simulink model "satellite3"  (R2025b)
settings: Solver=FixedStepAuto  StartTime=0.0  StopTime=100  FixedStep=dt  MinStep=0.0001  RelTol=1e-3
values from neighbouring files (symbols this model uses):
  A_mw = [ ... (first row only)    [init_params.m]
  A_w = [ ... (first row only)    [init_params.m]
  alpha1 = 0.1    [init_params.m]
  alpha2 = 0.1    [init_params.m]
  angle0 = eAR'    [init_params.m]
  area_d = 4    [init_params.m]
  area_m2 = 0.0127    [init_params.m]
  area_s = 2    [init_params.m]
  ARW_deg_per_sqrt_h = 0.01    [init_params.m]
  B_mw = [ ... (first row only)    [init_params.m]
  bat_bias_on = 0    [init_params.m]
  bat_bias_time = 0    [init_params.m]
  bat_bias_value = 0    [init_params.m]
  bat_cap_on = 0    [init_params.m]
  bat_cap_time = 0    [init_params.m]
  bat_cap_value = 1    [init_params.m]
  beta = 0.3    [init_params.m]
  beta1 = 0.01    [init_params.m]
  beta2 = 0.01    [init_params.m]
  bias0_deg_h = 0.01    [init_params.m]
  C_mw = [ ... (first row only)    [init_params.m]
  Cd = 2.2    [init_params.m]
  Cm = 0.01    [init_params.m]
  cmd_comm = 1    [init_params.m]
  comm_allow = 1    [init_params.m]
  cos_g_max = cos(gamma_max)    [init_params.m]
  Cr = 1.2    [init_params.m]
  cT_deg_on = 0    [init_params.m]
  cT_deg_time = 0    [init_params.m]
  cT_deg_value = 1    [init_params.m]
  cT_delay_on = 0    [init_params.m]
  cT_delay_time = 0    [init_params.m]
  cT_delay_value = 0    [init_params.m]
  cT_drop_on = 0    [init_params.m]
  cT_drop_time = 0    [init_params.m]
  cT_drop_value = 0    [init_params.m]
  cT_lock_on = 0    [init_params.m]
  cT_lock_time = 0    [init_params.m]
  d_c = 2e-5    (= 2e-05)    [init_params.m]
  d_f = 2e-5    (= 2e-05)    [init_params.m]
  D_max = 1    [init_params.m]
  D_thr = 0.4    [init_params.m]
  Delta_D = 0.001    [init_params.m]
  dP_th = 0.05    [init_params.m]
  dss_bias_on = 0    [init_params.m]
  dss_bias_time = 0    [init_params.m]
  dss_bias_value = [0;0;0]    [init_params.m]
  dss_delay_on = 0    [init_params.m]
  dss_delay_time = 0    [init_params.m]
  dss_delay_value = 0    [init_params.m]
  dss_drift_max = 0.1    [init_params.m]
  dss_drift_value = [0;0;0]    [init_params.m]
  dss_drop_on = 0    [init_params.m]
  dss_drop_time = 0    [init_params.m]
  dss_drop_value = [1;0;0]    [init_params.m]
  dss_lock_on = 0    [init_params.m]
  dss_lock_time = 0    [init_params.m]
  dt = 0.1    [init_params.m]
  earth_theta0 = 0    [init_params.m]
  epsilon = 0.01    [init_params.m]
  eT_deg_on = 0    [init_params.m]
  eT_deg_time = 0    [init_params.m]
  eT_deg_value = 1    [init_params.m]
  eT_delay_on = 0    [init_params.m]
  eT_delay_time = 0    [init_params.m]
  eT_delay_value = 0    [init_params.m]
  eT_drop_on = 0    [init_params.m]
  eT_drop_time = 0    [init_params.m]
  eT_drop_value = [0;0;0]    [init_params.m]
  eT_lock_on = 0    [init_params.m]
  eT_lock_time = 0    [init_params.m]
  eta = 0.7    [init_params.m]
  eta_buck = 0.9    [init_params.m]
  eta_et = 0.9    [init_params.m]
  eta_sspa = 0.35    [init_params.m]
  eta_twta = 0.35    [init_params.m]
  f = 2.2e9    (= 2200000000)    [init_params.m]
  f_n_hz = 400    [init_params.m]
  fov = 60*pi/180    (= 1.0471975512)    [init_params.m]
  g0 = 9.80665    [init_params.m]
  G0 = 1366.1    [init_params.m]
  G_sspa_dB = 20    [init_params.m]
  G_twta_dB = 20    [init_params.m]
  Gr_dB = 20    [init_params.m]
  Gt_dB = 3    [init_params.m]
  gyro_bias_on = 0    [init_params.m]
  gyro_bias_time = 0    [init_params.m]
  gyro_bias_value = [0;0;0]    [init_params.m]
  gyro_delay_on = 0    [init_params.m]
  gyro_delay_time = 0    [init_params.m]
  gyro_delay_value = 0    [init_params.m]
  gyro_drift_max = 0.1    [init_params.m]
  gyro_drift_value = [0;0;0]    [init_params.m]
  gyro_drop_on = 0    [init_params.m]
  gyro_drop_time = 0    [init_params.m]
  gyro_drop_value = [0;0;0]    [init_params.m]
  gyro_lock_on = 0    [init_params.m]
  gyro_lock_time = 0    [init_params.m]
  H = 50e3    (= 50000)    [init_params.m]
  h_max = Iw * rpm_max * sqrt(6)    [init_params.m]
  h_ref = 400e3    (= 400000)    [init_params.m]
  I_e = 11    [init_params.m]
  I_gate = 0.5    [init_params.m]
  I_triggle = 8    [init_params.m]
  i_w_max = 2    [init_params.m]
  i_w_min = -2    [init_params.m]
  initial_phase = 0    [init_params.m]
  Isp = 220    [init_params.m]
  Isp_et = 1500    [init_params.m]
  Iw = 0.02    [init_params.m]
  J2 = 1.08262668e-3    (= 0.00108262668)    [init_params.m]
  Jx = 10    [init_params.m]
  Jy = 12    [init_params.m]
  Jz = 8    [init_params.m]
  k_a = 4e-4    (= 0.0004)    [init_params.m]
  k_bias1_deg_h_per_C = 1    [init_params.m]
  k_bias2_deg_h_per_C = 0.0    (= 0)    [init_params.m]
  k_h = -0.05    [init_params.m]
  k_sf1_ppm = 1.0    (= 1)    [init_params.m]
  k_sf2_ppm = 0.0    (= 0)    [init_params.m]
  ... (+207 more)
libraries: matrix_library x25, simulink x14, nesl_utility x4, simulink_extras x3, fl_lib x3, ee_lib x1
(part 1 of 5)
settings Model: PauseTimes=2600  PacingRate=0.100000  Creator=NUAA  LastModifiedBy=NUAA
settings SolverCC: InitialStep=0.0001

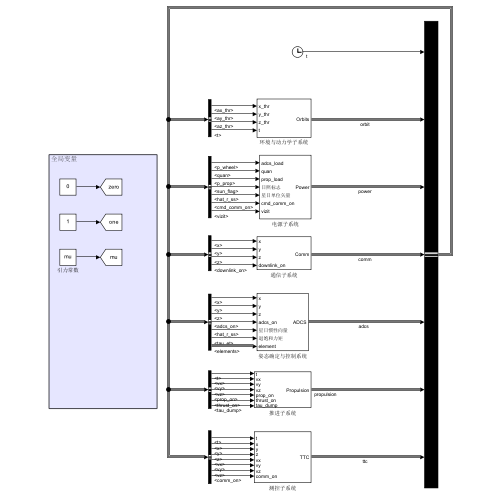
[thumbnail: Simulink's stored preview of the top-level diagram]
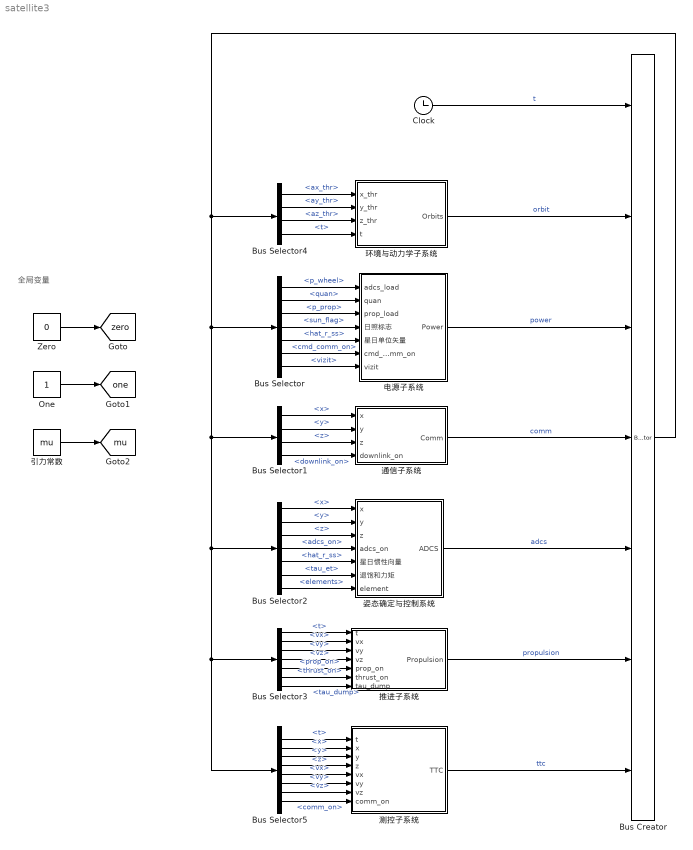
== system satellite3 ==
  note: 全局变量
  Bus Creator : BusCreator  Inputs=7  OutDataTypeStr=Bus: sat
  Bus Selector : BusSelector  OutputSignals=adcs.p_wheel,adcs.quan,propulsion.p_prop,orbit.sun_flag,orbit.hat_r_ss,ttc.cmd_comm_on,ttc.vizit
  Bus Selector1 : BusSelector  OutputSignals=orbit.states.x,orbit.states.y,orbit.states.z,ttc.downlink_on
  Bus Selector2 : BusSelector  OutputSignals=orbit.states.x,orbit.states.y,orbit.states.z,power.adcs_on,orbit.hat_r_ss,propulsion.tau_et,orbit.elements
  Bus Selector3 : BusSelector  OutputSignals=t,orbit.states.vx,orbit.states.vy,orbit.states.vz,power.prop_on,orbit.thrust_on,adcs.tau_dump
  Bus Selector4 : BusSelector  OutputSignals=propulsion.ax_thr,propulsion.ay_thr,propulsion.az_thr,t
  Bus Selector5 : BusSelector  OutputSignals=t,orbit.states.x,orbit.states.y,orbit.states.z,orbit.states.vx,orbit.states.vy,orbit.states.vz,power.comm_on
  Clock : Clock
  One : Constant  OutDataTypeStr=Inherit: Inherit via back propagation
  Zero : Constant  Value=0  OutDataTypeStr=Inherit: Inherit via back propagation
  姿态确定与控制系统 : Subsystem
  引力常数 : Constant  Value=mu  OutDataTypeStr=Inherit: Inherit via back propagation
  推进子系统 : Subsystem
  测控子系统 : Subsystem
  环境与动力学子系统 : Subsystem
  电源子系统 : Subsystem
  通信子系统 : Subsystem
  tag scope: mu=global, one=global, zero=global
  wires:
  Zero/1 -> [zero]
  One/1 -> [one]
  引力常数/1 -> [mu]
  环境与动力学子系统/1(Orbits) -> Bus Creator/2  "orbit"
  电源子系统/1(Power) -> Bus Creator/3  "power"
  Bus Creator/1 -> Bus Selector5/1, Bus Selector3/1, Bus Selector2/1, Bus Selector1/1, Bus Selector/1, Bus Selector4/1
  通信子系统/1(Comm) -> Bus Creator/4  "comm"
  姿态确定与控制系统/1(ADCS) -> Bus Creator/5  "adcs"
  Bus Selector/1 -> 电源子系统/1(adcs_load)  "<p_wheel>"
  Bus Selector/2 -> 电源子系统/2(quan)  "<quan>"
  Bus Selector1/1 -> 通信子系统/1(x)  "<x>"
  Bus Selector1/2 -> 通信子系统/2(y)  "<y>"
  Bus Selector1/3 -> 通信子系统/3(z)  "<z>"
  Bus Selector1/4 -> 通信子系统/4(downlink_on)  "<downlink_on>"
  Bus Selector2/1 -> 姿态确定与控制系统/1(x)  "<x>"
  Bus Selector2/2 -> 姿态确定与控制系统/2(y)  "<y>"
  Bus Selector2/3 -> 姿态确定与控制系统/3(z)  "<z>"
  Clock/1 -> Bus Creator/1  "t"
  Bus Selector2/4 -> 姿态确定与控制系统/4(adcs_on)  "<adcs_on>"
  Bus Selector3/1 -> 推进子系统/1(t)  "<t>"
  Bus Selector3/2 -> 推进子系统/2(vx)  "<vx>"
  Bus Selector3/3 -> 推进子系统/3(vy)  "<vy>"
  推进子系统/1(Propulsion) -> Bus Creator/6  "propulsion"
  Bus Selector/3 -> 电源子系统/3(prop_load)  "<p_prop>"
  Bus Selector3/5 -> 推进子系统/5(prop_on)  "<prop_on>"
  Bus Selector4/1 -> 环境与动力学子系统/1(x_thr)  "<ax_thr>"
  Bus Selector4/2 -> 环境与动力学子系统/2(y_thr)  "<ay_thr>"
  Bus Selector3/4 -> 推进子系统/4(vz)  "<vz>"
  Bus Selector4/3 -> 环境与动力学子系统/3(z_thr)  "<az_thr>"
  Bus Selector/4 -> 电源子系统/4(日照标志)  "<sun_flag>"
  Bus Selector4/4 -> 环境与动力学子系统/4(t)  "<t>"
  Bus Selector/5 -> 电源子系统/5(星日单位矢量)  "<hat_r_ss>"
  Bus Selector3/6 -> 推进子系统/6(thrust_on)  "<thrust_on>"
  Bus Selector2/5 -> 姿态确定与控制系统/5(星日惯性向量)  "<hat_r_ss>"
  测控子系统/1(TTC) -> Bus Creator/7  "ttc"
  Bus Selector5/2 -> 测控子系统/2(x)  "<x>"
  Bus Selector5/3 -> 测控子系统/3(y)  "<y>"
  Bus Selector5/5 -> 测控子系统/5(vx)  "<vx>"
  Bus Selector5/6 -> 测控子系统/6(vy)  "<vy>"
  Bus Selector5/8 -> 测控子系统/8(comm_on)  "<comm_on>"
  Bus Selector5/4 -> 测控子系统/4(z)  "<z>"
  Bus Selector5/1 -> 测控子系统/1(t)  "<t>"
  Bus Selector5/7 -> 测控子系统/7(vz)  "<vz>"
  Bus Selector3/7 -> 推进子系统/7(tau_dump)  "<tau_dump>"
  Bus Selector2/6 -> 姿态确定与控制系统/6(退饱和力矩)  "<tau_et>"
  Bus Selector2/7 -> 姿态确定与控制系统/7(element)  "<elements>"
  Bus Selector/6 -> 电源子系统/6(cmd_comm_on)  "<cmd_comm_on>"
  Bus Selector/7 -> 电源子系统/7(vizit)  "<vizit>"

== system satellite3/姿态确定与控制系统 ==
  x : Inport
  y : Inport  Port=2
  z : Inport  Port=3
  adcs_on : Inport  Port=4
  星日惯性向量 : Inport  Port=5
  退饱和力矩 : Inport  Port=6
  element : Inport  Port=7
  Mux : Mux  Inputs=3
  adcs : BusCreator  Inputs=5  OutDataTypeStr=Bus: adcs
  三轴PD控制器 : Subsystem
  三轴姿态动力学子系统 : Subsystem
      settings: PortSchema="{\"entries\":[{\"content\":{\"sides\":[{\"content\":{\"connectorIds\":[\"In1\",\"In2\",\"In3\"]},\"type\":\"ConnectorPlacement.EquallySpacedRectSide\",\"uuid\":\"b4e63c58-179c-42e3-802d-9c031f031a76\"},{\"content\":{\"connectorIds\":[\"Out1\",\"Out2\",\"Out3\",\"Out4\"],\"side\":\"RIGHT\"},\"type\":\"ConnectorPlacement.EquallySpacedRectSide\",\"uuid\":\"cea4ba66-c4d0-47a6-9ed8-1d5f6e65d5fe\"},{\"content\":{\"connectorIds\":[\"In4\"],\"side\":\"TOP\"},\"type\":\"ConnectorPlacement.EquallySpacedRectSide\",\"uuid\":\"baa71e33-906a-48b3-8a74-2d8b41e12ad9\"},{\"content\":{\"connectorIds\":[\"In5\",\"In6\"],\"side\":\"BOTTOM\"},\"type\":\"ConnectorPlacement.EquallySpacedRectSide\",\"uuid\":\"b6ab8a99-17e4-4d0c-a22a-7f74a164c022\"}]},\"type\":\"ConnectorPlacement.EquallySpacedConnector\",\"uuid\":\"2068c6e4-cb5a-485a-b5bc-bcb903ef601f\"}],\"packageUris\":[\"http://schema.mathworks.com/mf0/Connector/R2020b\"],\"version\":\"1.0\"}"
  向量模长-r_i : Subsystem
  期望四元数 : Constant  Value=QE
  重力梯度力矩 : Subsystem
      settings: PortSchema="{\"entries\":[{\"content\":{\"sides\":[{\"content\":{\"connectorIds\":[\"In1\",\"In2\"]},\"type\":\"ConnectorPlacement.EquallySpacedRectSide\",\"uuid\":\"5e08f9a5-0f22-478e-8a9e-735dc3411939\"},{\"content\":{\"connectorIds\":[\"Out1\",\"Out2\"],\"side\":\"RIGHT\"},\"type\":\"ConnectorPlacement.EquallySpacedRectSide\",\"uuid\":\"e11357c3-d338-4915-97ea-64fb65c259bd\"},{\"content\":{\"side\":\"TOP\"},\"type\":\"ConnectorPlacement.EquallySpacedRectSide\",\"uuid\":\"d2466a98-85a6-4c0d-931a-0ea5053455e9\"},{\"content\":{\"connectorIds\":[\"In3\"],\"side\":\"BOTTOM\"},\"type\":\"ConnectorPlacement.EquallySpacedRectSide\",\"uuid\":\"c799e970-0051-4874-a153-25b8e5bd94de\"}]},\"type\":\"ConnectorPlacement.EquallySpacedConnector\",\"uuid\":\"15237443-cc64-471d-b88e-214b003eddb8\"}],\"packageUris\":[\"http://schema.mathworks.com/mf0/Connector/R2020b\"],\"version\":\"1.0\"}"
  金字塔反作用轮组件 : Subsystem
  ADCS : Outport
  wires:
  三轴PD控制器/1(指令力矩) -> 金字塔反作用轮组件/1(指令力矩)
  金字塔反作用轮组件/1(反作用力矩) -> 三轴姿态动力学子系统/1(反作用力矩)
  三轴姿态动力学子系统/2(解算角速度) -> 三轴PD控制器/2(实际角速率)
  Mux/1 -> 重力梯度力矩/1(r_i)
  y/1 -> 向量模长-r_i/2(u1), Mux/2
  x/1 -> 向量模长-r_i/1(u0), Mux/1
  z/1 -> 向量模长-r_i/3(u2), Mux/3
  向量模长-r_i/1(|u|) -> 重力梯度力矩/2(|r_i|)
  重力梯度力矩/1(T_gg) -> 三轴姿态动力学子系统/3(重力梯度力矩)
  adcs/1 -> ADCS/1
  三轴姿态动力学子系统/1(解算四元数) -> adcs/2, 三轴PD控制器/1(实际四元数)  "quan"
  三轴姿态动力学子系统/3(欧拉数) -> adcs/3  "euler_angle"
  金字塔反作用轮组件/2(轮角动量) -> 三轴姿态动力学子系统/2(轮角动量)
  重力梯度力矩/2(r_o) -> 三轴姿态动力学子系统/5(hat_r_o)
  星日惯性向量/1 -> 三轴姿态动力学子系统/6(hat_ss_i)
  期望四元数/1 -> 三轴PD控制器/3(期望四元数)
  adcs_on/1 -> 三轴PD控制器/4(on)
  金字塔反作用轮组件/3(轮功耗) -> adcs/1  "p_wheel"
  金字塔反作用轮组件/4(wheel) -> adcs/4  "wheel"
  金字塔反作用轮组件/5(指令退饱和力矩) -> adcs/5  "tau_dump"
  退饱和力矩/1 -> 三轴姿态动力学子系统/4(退饱和力矩)
  element/1 -> 重力梯度力矩/3(element)

== system satellite3/推进子系统 ==
  note: 化学推进器 ：主要消耗推进剂，电功耗只体现在阀门/控制器，可设很小常数。
      | 电推进器 ：电功耗很大，推力很小。
  note: 1. 接收供电指令和点火指令。
      | 2. 计算实际推力 T_actual 。
      | 3. 根据 Isp 计算推进剂消耗，积分得到剩余推进剂质量 m_prop 。
      | 4. 用 四元数 把机体系推力方向旋转到惯性系，得到 F_ix, F_iy 。
      | 5. 输出推进加速度 a_thr_x, a_thr_y 给现有 Dynamics，并输出 P_thruster 给现有 Power。
  t : Inport
  vx : Inport  Port=2
  vy : Inport  Port=3
  vz : Inport  Port=4
  prop_on : Inport  Port=5
  thrust_on : Inport  Port=6
  tau_dump : Inport  Port=7
  Add : Sum  Inputs=+++
  Bus Creator : BusCreator  Inputs=5  OutDataTypeStr=Bus: propulsion
  Constant : Constant  Value=m-m0-m0_et
  Divide : Product  Inputs=/*
  Divide1 : Product  Inputs=/*
  Divide2 : Product  Inputs=*/
  Divide3 : Product  Inputs=/*
  Product : Product
  Product1 : Product
  Product2 : Product
  Scope : Scope
      settings: ActiveDisplayYMinimum=0.039953215564435186  ActiveDisplayYMaximum=0.0404210599200833  DataLoggingVariableName=ScopeData26
  Sum : Sum  Inputs=++|
  化推 : Subsystem
  化推功耗 : Switch  Criteria=u2 > Threshold  SaturateOnIntegerOverflow=off  InputSameDT=off
  向量模长-v : Subsystem
  推进功耗 : Constant  Value=P_prop
  电推 : Subsystem
  Propulsion : Outport
  wires:
  prop_on/1 -> 电推/1(prop_on), 化推/1(prop_on)  "电"
  thrust_on/1 -> 化推/2(thrust_on)  "推"
  vy/1 -> Divide1/2, 向量模长-v/2(u2)
  vx/1 -> Divide/2, 向量模长-v/1(u1)
  向量模长-v/1(|u|) -> Divide3/1, Divide/1, Divide1/1
  Constant/1 -> Add/3
  化推/2(left_fuel) -> Add/2
  Add/1 -> Divide2/2
  化推/1(T_act) -> Divide2/1, 化推功耗/2
  Divide/1 -> Product/2
  Divide2/1 -> Scope/1, Product2/1, Product1/1, Product/1
  Divide1/1 -> Product1/2
  推进功耗/1 -> 化推功耗/1
  [zero] -> 化推功耗/3
  Sum/1 -> Bus Creator/2  "p_prop"
  Product/1 -> Bus Creator/3  "ax_thr"
  Product1/1 -> Bus Creator/4  "ay_thr"
  Bus Creator/1 -> Propulsion/1
  vz/1 -> Divide3/2, 向量模长-v/3(u3)
  Product2/1 -> Bus Creator/5  "az_thr"
  Divide3/1 -> Product2/2
  化推功耗/1 -> Sum/2  "p_prop"
  电推/2(left_fuel) -> Add/1
  电推/3(P_et) -> Sum/1  "p_prop"
  tau_dump/1 -> 电推/2(退饱和指令力矩)
  电推/1(tau_et) -> Bus Creator/1  "tau_et"

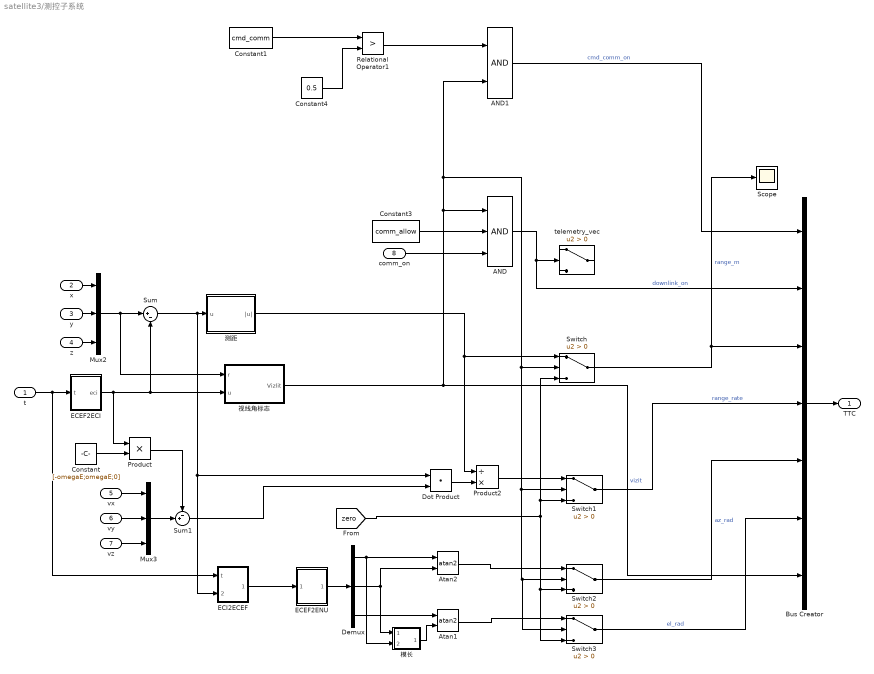
== system satellite3/测控子系统 ==
  t : Inport
  x : Inport  Port=2
  y : Inport  Port=3
  z : Inport  Port=4
  vx : Inport  Port=5
  vy : Inport  Port=6
  vz : Inport  Port=7
  comm_on : Inport  Port=8
  AND : Logic  Inputs=3  AllPortsSameDT=off  OutDataTypeStr=boolean
  AND1 : Logic  AllPortsSameDT=off  OutDataTypeStr=boolean
  Atan1 : Trigonometry  Operator=atan2
  Atan2 : Trigonometry  Operator=atan2
  Bus Creator : BusCreator  Inputs=7  OutDataTypeStr=Bus: ttc
  Constant : Constant  Value=[-omegaE;omegaE;0]
  Constant1 : Constant  Value=cmd_comm
  Constant3 : Constant  Value=comm_allow
  Constant4 : Constant  Value=0.5
  Demux : Demux  Outputs=3
  Dot Product : DotProduct  OutDataTypeStr=Inherit: Inherit via internal rule
  ECEF2ECI : Subsystem
  ECEF2ENU : Subsystem
  ECI2ECEF : Subsystem
  Mux2 : Mux  Inputs=3
  Mux3 : Mux  Inputs=3
  Product : Product
  Product2 : Product  Inputs=/*
  Relational Operator1 : RelationalOperator  Operator=>  OutDataTypeStr=boolean  RndMeth=Simplest  InputSameDT=off
  Scope : Scope
      settings: ActiveDisplayYMinimum=-889765.13346337143  ActiveDisplayYMaximum=8.0078862011703448E+6  DataLoggingVariableName=ScopeData20
  Sum : Sum  Inputs=|+-
  Sum1 : Sum  Inputs=-+|
  Switch{,1..3} (4 alike) : Switch  Criteria=u2 > Threshold  SaturateOnIntegerOverflow=off  InputSameDT=off
  telemetry_vec : Switch  Criteria=u2 > Threshold  SaturateOnIntegerOverflow=off  InputSameDT=off
  模长 : Subsystem
  测距 : Subsystem
  视线角标志 : Subsystem
  TTC : Outport
  wires:
  视线角标志/1(Vizlit) -> Bus Creator/7, AND1/2, Switch3/2, Switch2/2, Switch1/2, Switch/2, AND/1  "vizit"
  测距/1(|u|) -> Switch/1, Product2/1
  Sum1/1 -> Dot Product/2
  Dot Product/1 -> Product2/2
  Product2/1 -> Switch1/1
  Atan2/1 -> Switch2/1
  Constant3/1 -> AND/2
  comm_on/1 -> AND/3
  AND/1 -> Bus Creator/2, telemetry_vec/2  "downlink_on"
  [zero] -> Switch1/3, Switch/3, Switch3/3, Switch2/3
  Switch/1 -> Scope/1, Bus Creator/3  "range_m"
  Switch1/1 -> Bus Creator/4  "range_rate"
  Switch2/1 -> Bus Creator/5  "az_rad"
  Constant1/1 -> Relational Operator1/1
  AND1/1 -> Bus Creator/1  "cmd_comm_on"
  Constant4/1 -> Relational Operator1/2
  Relational Operator1/1 -> AND1/1
  Bus Creator/1 -> TTC/1
  t/1 -> ECI2ECEF/1(t), ECEF2ECI/1(t)
  x/1 -> Mux2/1
  y/1 -> Mux2/2
  z/1 -> Mux2/3
  Mux2/1 -> 视线角标志/1(r), Sum/1
  ECEF2ECI/1(eci) -> Product/1, 视线角标志/2(u), Sum/2
  Sum/1 -> ECI2ECEF/2(In1), Dot Product/1, 测距/1(u)
  vx/1 -> Mux3/1
  vy/1 -> Mux3/2
  vz/1 -> Mux3/3
  Constant/1 -> Product/2
  Mux3/1 -> Sum1/2
  Product/1 -> Sum1/1
  ECI2ECEF/1(ecef) -> ECEF2ENU/1(ecef)
  ECEF2ENU/1(enu) -> Demux/1
  Demux/1 -> 模长/2(u2), Atan2/1
  Demux/2 -> 模长/1(u1), Atan2/2
  Demux/3 -> Atan1/1
  模长/1(|u|) -> Atan1/2
  Atan1/1 -> Switch3/1
  Switch3/1 -> Bus Creator/6  "el_rad"

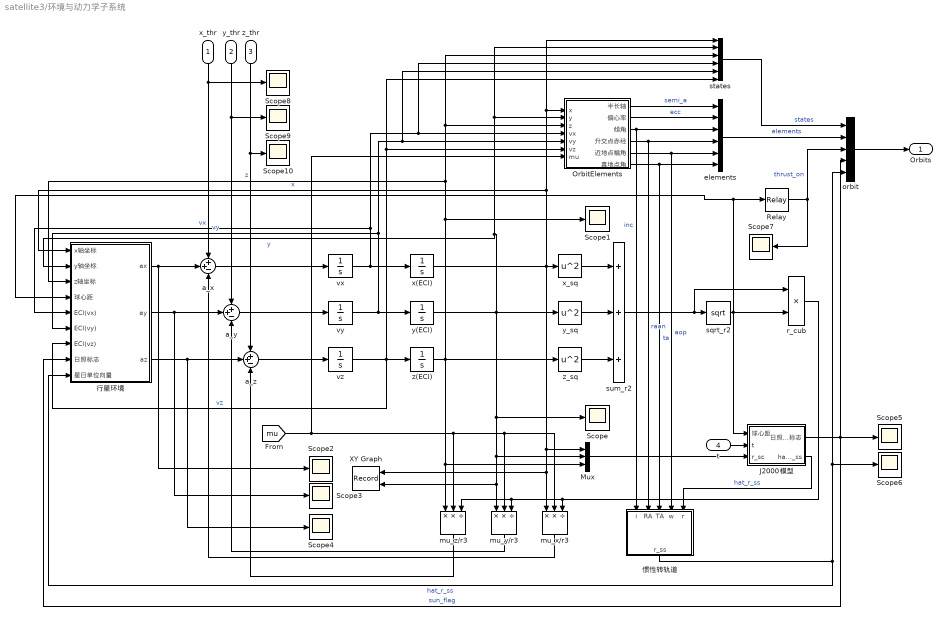
== system satellite3/环境与动力学子系统 ==
  x_thr : Inport
  y_thr : Inport  Port=2
  z_thr : Inport  Port=3
  t : Inport  Port=4
  J2000模型 : Subsystem
  Mux : Mux  Inputs=3
  OrbitElements : Subsystem
  Relay : Relay  OnSwitchValue=r_ref+1e3  OffSwitchValue=r_ref  OnOutputValue=0  OffOutputValue=1  OutDataTypeStr=boolean
  Scope{,1..10} (11 alike) : Scope
      Scope settings: ActiveDisplayYMinimum=-8.9402554358248618E+6  ActiveDisplayYMaximum=8.80467459081228E+6
      Scope1 settings: ActiveDisplayYMinimum=-1  ActiveDisplayYMaximum=1
      Scope10 settings: ActiveDisplayYMinimum=-1  ActiveDisplayYMaximum=1  DataLoggingVariableName=ScopeData25
      Scope2 settings: ActiveDisplayYMinimum=-0.013724283489942623  ActiveDisplayYMaximum=0.013844629667354235  DataLoggingVariableName=ScopeData2
      Scope3 settings: ActiveDisplayYMinimum=-0.013784437757224171  ActiveDisplayYMaximum=0.013784949077631064  DataLoggingVariableName=ScopeData3
      Scope4 settings: ActiveDisplayYMinimum=-5.0430131814522649E-6  ActiveDisplayYMaximum=5.7232220678912172E-7  DataLoggingVariableName=ScopeData4
      Scope5 settings: ActiveDisplayYMinimum=-1  ActiveDisplayYMaximum=1  DataLoggingVariableName=ScopeData10
      Scope6 settings: ActiveDisplayYMinimum=-1  ActiveDisplayYMaximum=1  DataLoggingVariableName=ScopeData17
      Scope7 settings: ActiveDisplayYMinimum=0.88223040201005021  ActiveDisplayYMaximum=1.1253316520100503  DataLoggingVariableName=ScopeData18
      Scope8 settings: ActiveDisplayYMinimum=-1  ActiveDisplayYMaximum=1  DataLoggingVariableName=ScopeData21
      Scope9 settings: ActiveDisplayYMinimum=-1  ActiveDisplayYMaximum=1  DataLoggingVariableName=ScopeData22
  XY Graph : Record  NumPorts=2.0  FileSettingsInternal="{\"entries\":[{\"content\":{\"excelSettings\":{\"content\":{},\"type\":\"Streamout.ExcelSettings\"},\"parquetSettings\":{\"content\":{},\"type\":\"Streamout.ParquetSettings\"}},\"type\":\"Streamout.FileSettingStorage\",\"uuid\":\"\"}],\"packageUris\":[\"http:\\/\\/schema.mathworks.com\\/mf0\\/streamout_blocks\\/R2020a\"],\"version\":\"1.0\"}"  FrameSettings=[0, 0]  Layout=[1 1]  SignalsInternal="{\"entries\":[{\"content\":{\"signals\":[{\"content\":{\"blockPath\":[],\"dimensions\":[1],\"domain\":\"\",\"lineColor\":\"#a2142f\",\"plots\":[ 1 ],\"port\":1,\"sid\":[\"\"],\"signalID\":1,\"signalName\":\"x\"},\"type\":\"RecordBlkView.Signal\",\"uuid\":\"\"},{\"content\":{\"blockPath\":[],\"dimensions\":[1],\"domain\":\"\",\"lineColor\":\"#139fff\",\"plots\":[ 1 ],\"port\":2,\"sid\":[\"\"],\"signalID\":2,\"signalName\":\"y\"},\"type\":\"RecordBlkView.Signal\",\"uuid\":\"\"}]},\"type\":\"RecordBlkView.InputSignals\",\"uuid\":\"\"}],\"packageUris\":[\"http:\\/\\/schema.mathworks.com\\/mf0\\/streamout_blocks\\/R2020a\"],\"version\":\"1.0\"}"  VisualizationBindings="{\"xyplotplugin\":{\"info\":[{\"series\":[{\"bindingParametersList\":[{\"parameter\":\"X-Axis\",\"signalID\":1,\"signalName\":\"x\"},{\"parameter\":\"Y-Axis\",\"signalID\":2,\"signalName\":\"y\"}],\"seriesID\":0}],\"subplotID\":1}]}}"  CompatibilityTag=XY
  a_x : Sum  Inputs=++-
  a_y : Sum  Inputs=++-
  a_z : Sum  Inputs=++-
  elements : BusCreator  Inputs=6  OutDataTypeStr=Bus: elements
  mu_x/r3 : Product  Inputs=**/
  mu_y/r3 : Product  Inputs=**/
  mu_z/r3 : Product  Inputs=**/
  orbit : BusCreator  Inputs=5  OutDataTypeStr=Bus: orbit
  r_cub : Product
  sqrt_r2 : Sqrt
  states : BusCreator  Inputs=6  OutDataTypeStr=Bus: states
  sum_r2 : Sum  Inputs=+++
  vx : Integrator  InitialCondition=vx0
  vy : Integrator  InitialCondition=vy0
  vz : Integrator  InitialCondition=vz0
  x(ECI) : Integrator  InitialCondition=x0
  x_sq : Math  Operator=square
  y(ECI) : Integrator  InitialCondition=y0
  y_sq : Math  Operator=square
  z(ECI) : Integrator  InitialCondition=z0
  z_sq : Math  Operator=square
  惯性转轨道 : MATLAB Function  TreatAsAtomicUnit=on
  行星环境 : Subsystem
  Orbits : Outport
  wires:
  vx/1 -> states/4, OrbitElements/4(vx), 行星环境/5(ECI(vx)), x(ECI)/1  "vx"
  vy/1 -> states/5, OrbitElements/5(vy), 行星环境/6(ECI(vy)), y(ECI)/1  "vy"
  vz/1 -> OrbitElements/6(vz), states/6, 行星环境/7(ECI(vz)), z(ECI)/1  "vz"
  y(ECI)/1 -> y_sq/1, states/2, OrbitElements/2(y), 行星环境/2(y轴坐标), XY Graph/2, mu_y/r3/1, Mux/2, Scope/1  "y"
  x_sq/1 -> sum_r2/1
  y_sq/1 -> sum_r2/2
  z_sq/1 -> sum_r2/3
  sum_r2/1 -> r_cub/1, sqrt_r2/1
  sqrt_r2/1 -> 行星环境/4(球心距), Relay/1, J2000模型/1(球心距), r_cub/2
  [mu] -> OrbitElements/7(mu), mu_x/r3/2, mu_y/r3/2, mu_z/r3/2
  r_cub/1 -> mu_x/r3/3, mu_y/r3/3, mu_z/r3/3
  mu_z/r3/1 -> a_z/3
  a_z/1 -> vz/1
  a_y/1 -> vy/1
  mu_y/r3/1 -> a_y/3
  mu_x/r3/1 -> a_x/3
  x(ECI)/1 -> XY Graph/1, mu_x/r3/1, Mux/1, x_sq/1, states/1, OrbitElements/1(x), 行星环境/1(x轴坐标)  "x"
  z(ECI)/1 -> z_sq/1, mu_z/r3/1, Mux/3, 行星环境/3(z轴坐标), states/3, OrbitElements/3(z), Scope1/1  "z"
  行星环境/1(ax) -> a_x/2, Scope2/1
  行星环境/2(ay) -> a_y/2, Scope3/1
  行星环境/3(az) -> a_z/2, Scope4/1
  a_x/1 -> vx/1
  OrbitElements/1(半长轴) -> elements/1  "semi_a"
  OrbitElements/2(偏心率) -> elements/2  "ecc"
  OrbitElements/3(倾角) -> elements/3, 惯性转轨道/1(i)  "inc"
  OrbitElements/4(升交点赤经) -> elements/4, 惯性转轨道/2(RA)  "raan"
  OrbitElements/5(近地点幅角) -> 惯性转轨道/4(w), elements/5  "aop"
  OrbitElements/6(真地点角) -> 惯性转轨道/3(TA), elements/6  "ta"
  elements/1 -> orbit/2  "elements"
  states/1 -> orbit/1  "states"
  orbit/1 -> Orbits/1
  x_thr/1 -> a_x/1, Scope8/1
  y_thr/1 -> Scope9/1, a_y/1
  Relay/1 -> Scope7/1, orbit/3  "thrust_on"
  z_thr/1 -> Scope10/1, a_z/1
  t/1 -> J2000模型/2(t)
  Mux/1 -> J2000模型/3(r_sc)
  J2000模型/1(日照标志) -> Scope5/1, orbit/4, 行星环境/8(日照标志)  "sun_flag"
  惯性转轨道/1(r_ss) -> orbit/5, Scope6/1, 行星环境/9(星日单位向量)  "hat_r_ss"
  J2000模型/2(hat_r_ss) -> 惯性转轨道/5(r)  "hat_r_ss"

== system satellite3/电源子系统 ==
  adcs_load : Inport
  quan : Inport  Port=2
  prop_load : Inport  Port=3
  日照标志 : Inport  Port=4
  星日单位矢量 : Inport  Port=5
  cmd_comm_on : Inport  Port=6
  vizit : Inport  Port=7
  Add : Sum  Inputs=++++
  Scope : Scope  NumInputPorts=3
      settings: ActiveDisplayYMinimum=-17.3265289803657  ActiveDisplayYMaximum=40.84827911882865  DataLoggingVariableName=ScopeData48
  power : BusCreator  Inputs=4  OutDataTypeStr=Bus: power
  充电调节器 : Subsystem
      settings: PortSchema="{\"entries\":[{\"content\":{\"sides\":[{\"content\":{},\"type\":\"ConnectorPlacement.EquallySpacedRectSide\",\"uuid\":\"1ee7afef-72a2-44d7-b1fe-f775c1bd2fb5\"},{\"content\":{\"connectorIds\":[\"In3\"],\"side\":\"RIGHT\"},\"type\":\"ConnectorPlacement.EquallySpacedRectSide\",\"uuid\":\"a705df99-5add-4aef-8a58-2d39c82bf6d7\"},{\"content\":{\"connectorIds\":[\"Out1\"],\"side\":\"TOP\"},\"type\":\"ConnectorPlacement.EquallySpacedRectSide\",\"uuid\":\"759de5c5-d633-4c5d-bf74-673abcd24ad6\"},{\"content\":{\"connectorIds\":[\"In1\",\"In2\"],\"side\":\"BOTTOM\"},\"type\":\"ConnectorPlacement.EquallySpacedRectSide\",\"uuid\":\"f7dc8a63-c562-404b-8603-e7c277e9b032\"}]},\"type\":\"ConnectorPlacement.EquallySpacedConnector\",\"uuid\":\"7ef34a9a-0568-4899-98ec-73e8b4fd5653\"}],\"packageUris\":[\"http://schema.mathworks.com/mf0/Connector/R2020b\"],\"version\":\"1.0\"}"
  太阳能板 : Subsystem
      settings: PortSchema="{\"entries\":[{\"content\":{\"sides\":[{\"content\":{\"connectorIds\":[\"In1\",\"In2\",\"In3\"]},\"type\":\"ConnectorPlacement.EquallySpacedRectSide\",\"uuid\":\"5bc779c2-c30f-4cae-b4e1-f2edac4125bf\"},{\"content\":{\"connectorIds\":[\"Out1\",\"Out2\",\"Out3\"],\"side\":\"RIGHT\"},\"type\":\"ConnectorPlacement.EquallySpacedRectSide\",\"uuid\":\"cdc54232-7dcb-45bf-9570-abbf77ba5ff8\"},{\"content\":{\"connectorIds\":[\"In4\",\"In5\",\"In6\"],\"side\":\"TOP\"},\"type\":\"ConnectorPlacement.EquallySpacedRectSide\",\"uuid\":\"7ae4bd94-3445-4ae2-aeac-bc49ea099582\"},{\"content\":{\"side\":\"BOTTOM\"},\"type\":\"ConnectorPlacement.EquallySpacedRectSide\",\"uuid\":\"0e5ffc09-da69-4730-b459-bd286bf114a0\"}]},\"type\":\"ConnectorPlacement.EquallySpacedConnector\",\"uuid\":\"4dec81bf-3de5-48e4-88d8-77ff2b0205f0\"}],\"packageUris\":[\"http://schema.mathworks.com/mf0/Connector/R2020b\"],\"version\":\"1.0\"}"
  姿态确认与控制功耗 : Subsystem
  平台常开负载功耗 : Constant  Value=P_base
  推进子系统功耗 : Subsystem
  蓄电池组 : Subsystem
      settings: PortSchema="{\"entries\":[{\"content\":{\"sides\":[{\"content\":{},\"type\":\"ConnectorPlacement.EquallySpacedRectSide\",\"uuid\":\"7e7ce6a8-f422-4b44-b417-981bf143e596\"},{\"content\":{\"connectorIds\":[\"Out1\",\"Out2\"],\"side\":\"RIGHT\"},\"type\":\"ConnectorPlacement.EquallySpacedRectSide\",\"uuid\":\"32e18879-bd9f-43be-9339-7cab6907b877\"},{\"content\":{\"connectorIds\":[\"Out3\"],\"side\":\"TOP\"},\"type\":\"ConnectorPlacement.EquallySpacedRectSide\",\"uuid\":\"64b37c81-2d28-4322-9005-45a88751c011\"},{\"content\":{\"connectorIds\":[\"In1\"],\"side\":\"BOTTOM\"},\"type\":\"ConnectorPlacement.EquallySpacedRectSide\",\"uuid\":\"597055be-0b91-4221-a6e9-97960dc29d81\"}]},\"type\":\"ConnectorPlacement.EquallySpacedConnector\",\"uuid\":\"41982541-c784-41b5-be8a-a88d5d627e5c\"}],\"packageUris\":[\"http://schema.mathworks.com/mf0/Connector/R2020b\"],\"version\":\"1.0\"}"
  通信子系统功耗 : Subsystem
  Power : Outport
  wires:
  蓄电池组/1(V_batt) -> 太阳能板/4(V_batt)
  日照标志/1 -> 太阳能板/1(日照标志), 通信子系统功耗/3(sunlit)
  通信子系统功耗/1(comm_on) -> power/3  "comm_on"
  通信子系统功耗/2(通信功耗) -> Add/2, Scope/2
  太阳能板/3(非欠压) -> 通信子系统功耗/4(not_shed), 推进子系统功耗/3(not_shed), 姿态确认与控制功耗/3(not_shed)
  太阳能板/2(负载电流) -> 充电调节器/1(负载电流)
  vizit/1 -> 通信子系统功耗/2(Vizlit)  "vizlit"
  cmd_comm_on/1 -> 通信子系统功耗/5(cmd_comm_on)
  蓄电池组/3(SOC) -> 充电调节器/3(荷电状态), 姿态确认与控制功耗/1(SOC), power/1, 通信子系统功耗/1(SOC), 推进子系统功耗/1(SOC)  "soc"
  蓄电池组/2(电流差) -> 太阳能板/5(电流差)
  adcs_load/1 -> 姿态确认与控制功耗/2(adcs_load)
  prop_load/1 -> 推进子系统功耗/2(prop_load)
  姿态确认与控制功耗/1(adcs_on) -> power/2  "adcs_on"
  姿态确认与控制功耗/2(P_adcs) -> Scope/1, Add/1
  平台常开负载功耗/1 -> Add/4
  推进子系统功耗/2(prop_on) -> power/4  "prop_on"
  推进子系统功耗/1(P_prop) -> Scope/3, Add/3
  power/1 -> Power/1
  Add/1 -> 太阳能板/6(P_load)
  quan/1 -> 太阳能板/2(q)
  星日单位矢量/1 -> 太阳能板/3(星日单位矢量)
  太阳能板/1(蓄电池充电电流) -> 充电调节器/2(太阳能电池电流)
  充电调节器/1(净充电电流) -> 蓄电池组/1(净充电电流)

== system satellite3/通信子系统 ==
  note: 链路功耗加了，发射功耗还未接入
  note: 通信链可用标志
  note: 接收功率
  note: 信噪比
  note: 把姿态误差引入通信天线增益
      | 引入地面站可见性（地球遮挡）
      | 通信成功 → 数据量积分（任务完成度）
      | 通信失败 → 自动进入安全模式
      | 多地面站切换（Switch + 几何判断）
  note: 如果后面想考虑姿态误差，
      | 只需要在Gt上再减一个pointing loss。
  note: 自由空间路径损耗
      | $\text{FSPL(dBW)}=20\log_{10}{(\frac{4\pi r f}{c})}$
  note: 后续可以改成与地面站的距离
  note: 后续可以添加固放和行波管
  x : Inport
  y : Inport  Port=2
  z : Inport  Port=3
  downlink_on : Inport  Port=4
  10dB : Constant
  20 : Gain  Gain=20
  4pi rf/c : Gain  Gain=4*pi*f
  > : RelationalOperator  Operator=>  OutDataTypeStr=boolean  RndMeth=Simplest  InputSameDT=off
  AND : Logic  AllPortsSameDT=off  OutDataTypeStr=boolean
  Add : Sum  Inputs=-+++
  Constant : Constant  Value=R_data
  Integrator : Integrator  LimitOutput=on  UpperSaturationLimit=1e7  LowerSaturationLimit=0
  Log_10 : Math  Operator=log10
  N_dBW : Constant  Value=Noise_dBW
  SSPA : Subsystem
  Sum : Sum  Inputs=|-+
  Switch : Switch  Criteria=u2 > Threshold  SaturateOnIntegerOverflow=off  InputSameDT=off
  TWTA : Subsystem
  comm : BusCreator  Inputs=4  OutDataTypeStr=Bus: comm
  data_downlinked : Scope
      settings: DataLoggingVariableName=ScopeData11
  发射功率 : Constant  Commented=on  Value=Pt_dBW
  向量模长-r : Subsystem
  地面站天线 : Constant  Value=Gr_dB
  星上天线 : Constant  Value=Gt_dB
  Comm : Outport
  wires:
  x/1 -> 向量模长-r/1(u1)
  y/1 -> 向量模长-r/2(u2)
  z/1 -> 向量模长-r/3(u3)
  向量模长-r/1(|u|) -> 4pi rf/c/1
  4pi rf/c/1 -> Log_10/1
  Log_10/1 -> 20/1
  20/1 -> comm/3, Add/1, Sum/2  "FSPL_dB"
  星上天线/1 -> Add/3
  地面站天线/1 -> Add/4
  Add/1 -> comm/4  "Pr_dBW"
  Sum/1 -> comm/2, >/1  "SNR_dB"
  N_dBW/1 -> Sum/1
  10dB/1 -> >/2
  AND/1 -> Switch/2, comm/1  "link_ok"
  >/1 -> AND/2
  comm/1 -> Comm/1
  downlink_on/1 -> TWTA/1(tx_on), SSPA/1(tx_on), AND/1
  SSPA/1(Pt_dBW) -> Add/2
  [zero] -> Switch/3
  Constant/1 -> Switch/1
  Switch/1 -> Integrator/1
  Integrator/1 -> data_downlinked/1

== system satellite3/姿态确定与控制系统/三轴PD控制器 ==
  note: 在 当前实际姿态 基础上进行的旋转 $Q_e$$ ，使得它叠加在 $Q_a$$ 之后，能够达到期望姿态 $Q_d$$ 。
      | $1:Q_a \otimes Q_e=Q_d \\ 2:Q_a^{-1} \otimes (Q_a \otimes Q_e)=Q_a^{-1} \otimes Q_d \\ 3:Q_e = Q_a^{-1} \otimes Q_d \\ 4:Q_e = Q_a^{*} \otimes Q_d$
  note: 姿态误差限幅，防止大误差时控制器给出不合理力矩
  实际四元数 : Inport
  实际角速率 : Inport  Port=2
  期望四元数 : Inport  Port=3
  on : Inport  Port=4
  Demux : Demux
  Mux : Mux  Inputs=3
  Product : Product
  Product1 : Product
  Relay(qe0) : Relay  OffOutputValue=-1
  Scope : Scope
      settings: ActiveDisplayYMinimum=-0.83029524631328933  ActiveDisplayYMaximum=3.1480849645197186  DataLoggingVariableName=ScopeData32
  Sum1 : Sum  Inputs=|+-
  Switch : Switch  Criteria=u2 > Threshold  SaturateOnIntegerOverflow=off  InputSameDT=off
  sign(q0) : Signum
  共轭 : Subsystem
  四元数乘法 : Subsystem
  四元数归一化 : Subsystem
  姿态控制器-微分 : Gain  Gain=Kd
  姿态控制器-比例 : Gain  Gain=Kp
  指令力矩 : Outport
  wires:
  Product/1 -> 姿态控制器-比例/1
  姿态控制器-比例/1 -> Sum1/1
  姿态控制器-微分/1 -> Sum1/2
  期望四元数/1 -> 四元数归一化/1(In1)
  实际四元数/1 -> 共轭/1(u)
  四元数乘法/1(四元数旋转偏差) -> Demux/1
  Demux/1 -> Relay(qe0)/1
  Demux/2 -> Mux/1
  Demux/3 -> Mux/2
  Demux/4 -> Mux/3
  Mux/1 -> Product/2
  Relay(qe0)/1 -> Product/1
  实际角速率/1 -> 姿态控制器-微分/1
  共轭/1(u^-1) -> 四元数乘法/1(Q1)
  on/1 -> Product1/2
  四元数归一化/1(Out1) -> 四元数乘法/2(Q2)
  Sum1/1 -> 指令力矩/1, Product1/1
  Product1/1 -> Scope/1

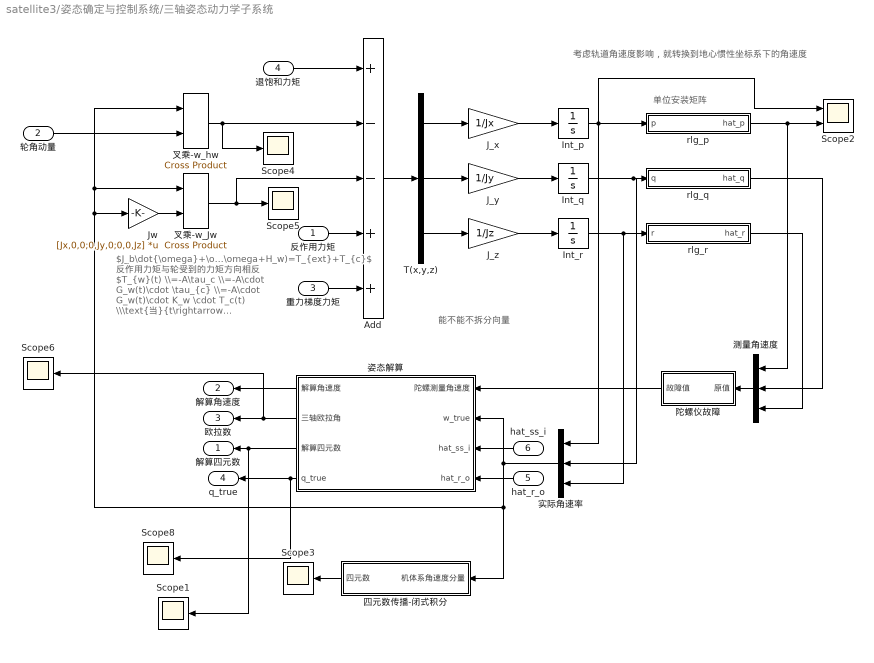
== system satellite3/姿态确定与控制系统/三轴姿态动力学子系统 ==
  note: $J_b\dot{\omega}+\omega\times(J_b\omega+H_w)=T_{ext}+T_{c}$
      | 反作用力矩与轮受到的力矩方向相反
      | $T_{w}(t) \\=-A\tau_c \\=-A\cdot G_w(t)\cdot \tau_{c} \\=-A\cdot G_w(t)\cdot K_w \cdot T_c(t) \\\text{当}{t\rightarrow t_s},G_w(t)=1,T_w(t)=-T_c(t)$
  note: 考虑轨道角速度影响，就转换到地心惯性坐标系下的角速度
  note: 能不能不拆分向量
  note: 单位安装矩阵
  反作用力矩 : Inport
  轮角动量 : Inport  Port=2
  重力梯度力矩 : Inport  Port=3
  退饱和力矩 : Inport  Port=4
  hat_r_o : Inport  Port=5
  hat_ss_i : Inport  Port=6
  Add : Sum  Inputs=+--++
  Int_p : Integrator  InitialCondition=w0(1)  LimitOutput=on  UpperSaturationLimit=p_sat*pi/180  LowerSaturationLimit=-10*pi/180
  Int_q : Integrator  InitialCondition=w0(2)  LimitOutput=on  UpperSaturationLimit=10*pi/180  LowerSaturationLimit=-10*pi/180
  Int_r : Integrator  InitialCondition=w0(3)  LimitOutput=on  UpperSaturationLimit=10*pi/180  LowerSaturationLimit=-10*pi/180
  J_x : Gain  Gain=1/Jx
  J_y : Gain  Gain=1/Jy
  J_z : Gain  Gain=1/Jz
  Jw : Gain  Gain=[Jx,0,0;0,Jy,0;0,0,Jz]  Multiplication=Matrix(K*u)
  Scope{1,3..6,8} (6 alike) : Scope
      Scope1 settings: ActiveDisplayYMinimum=-0.82477001832836239  ActiveDisplayYMaximum=0.987415638960409  DataLoggingVariableName=ScopeData8
      Scope3 settings: ActiveDisplayYMinimum=-0.607859112920923  ActiveDisplayYMaximum=1.0348923894829236  DataLoggingVariableName=ScopeData8
      Scope4 settings: ActiveDisplayYMinimum=-0.00074445474291978057  ActiveDisplayYMaximum=0.00081473788246158054  DataLoggingVariableName=ScopeData23
      Scope5 settings: ActiveDisplayYMinimum=-6.9419152004580546E-8  ActiveDisplayYMaximum=8.6121465383319188E-8  DataLoggingVariableName=ScopeData24
      Scope6 settings: ActiveDisplayYMinimum=-5.13179233941835  ActiveDisplayYMaximum=5.9674363348372523  DataLoggingVariableName=ScopeData31
      Scope8 settings: ActiveDisplayYMinimum=-1.164089564599627  ActiveDisplayYMaximum=1.0182326383526819  DataLoggingVariableName=ScopeData33
  Scope2 : Scope  NumInputPorts=2
      settings: ActiveDisplayYMinimum=-1.1823301841470205E-6  ActiveDisplayYMaximum=2.0642729555703557E-6  DataLoggingVariableName=ScopeData6
  T(x,y,z) : Demux  Outputs=3
  rlg_p : Subsystem
  rlg_q : Subsystem
  rlg_r : Subsystem
  叉乘-w_Jw : matrix_library/Cross Product
  叉乘-w_hw : matrix_library/Cross Product
  四元数传播-闭式积分 : Subsystem
  姿态解算 : Subsystem
  实际角速率 : Mux  Inputs=3
  测量角速度 : Mux  Inputs=3
  陀螺仪故障 : Subsystem
  解算四元数 : Outport
  解算角速度 : Outport  Port=2
  欧拉数 : Outport  Port=3
  q_true : Outport  Port=4
  wires:
  Add/1 -> T(x,y,z)/1
  叉乘-w_hw/1 -> Scope4/1, Add/2
  轮角动量/1 -> 叉乘-w_hw/2
  反作用力矩/1 -> Add/4
  J_z/1 -> Int_r/1
  T(x,y,z)/1 -> J_x/1
  J_y/1 -> Int_q/1
  T(x,y,z)/2 -> J_y/1
  J_x/1 -> Int_p/1
  T(x,y,z)/3 -> J_z/1
  Int_p/1 -> 实际角速率/1, Scope2/1, rlg_p/1(p)
  Int_q/1 -> 实际角速率/2, rlg_q/1(q)
  Int_r/1 -> 实际角速率/3, rlg_r/1(r)
  Jw/1 -> 叉乘-w_Jw/2
  叉乘-w_Jw/1 -> Scope5/1, Add/3
  重力梯度力矩/1 -> Add/5
  rlg_p/1(hat_p) -> 测量角速度/1, Scope2/2
  rlg_q/1(hat_q) -> 测量角速度/2
  rlg_r/1(hat_r) -> 测量角速度/3
  四元数传播-闭式积分/1(四元数) -> Scope3/1
  姿态解算/2(三轴欧拉角) -> Scope6/1, 欧拉数/1
  姿态解算/1(解算角速度) -> 解算角速度/1
  姿态解算/3(解算四元数) -> 解算四元数/1, Scope1/1
  姿态解算/4(q_true) -> q_true/1, Scope8/1
  实际角速率/1 -> 叉乘-w_hw/1, 叉乘-w_Jw/1, Jw/1, 四元数传播-闭式积分/1(机体系角速度分量), 姿态解算/2(w_true)
  测量角速度/1 -> 陀螺仪故障/1(原值)
  hat_r_o/1 -> 姿态解算/4(hat_r_o)
  hat_ss_i/1 -> 姿态解算/3(hat_ss_i)
  退饱和力矩/1 -> Add/1
  陀螺仪故障/1(故障值) -> 姿态解算/1(陀螺测量角速度)

== system satellite3/姿态确定与控制系统/向量模长-r_i ==
  u0 : Inport
  u1 : Inport  Port=2
  u2 : Inport  Port=3
  Add : Sum  Inputs=3
  Sqrt : Sqrt
  Square : Math  Operator=square
  Square1 : Math  Operator=square
  Square2 : Math  Operator=square
  |u| : Outport
  wires:
  u0/1 -> Square/1
  u1/1 -> Square1/1
  u2/1 -> Square2/1
  Square/1 -> Add/1
  Square1/1 -> Add/2
  Square2/1 -> Add/3
  Add/1 -> Sqrt/1
  Sqrt/1 -> |u|/1

== system satellite3/姿态确定与控制系统/重力梯度力矩 ==
  note: $\text{T}_{gg}=3\frac{\mu}{r^5}\hat{r}_B\times (J\hat{r}_B)$
  r_i : Inport
  |r_i| : Inport  Port=2
  element : Inport  Port=3
  Bus Selector : BusSelector  OutputSignals=inc,raan,ta,aop
  Constant : Constant  Value=5
  Divide : Product  Inputs=/*
  Gain : Gain  Gain=3
  Pow : Math  Operator=pow  OutputSignalType=real  RndMeth=Zero
  Product : Product  Multiplication=Matrix(*)
  Product1 : Product
  卫星对角转动惯量 : Constant  Value=[Jx,0,0;0,Jy,0;0,0,Jz]
  叉乘-r_Jr : matrix_library/Cross Product
  地心转轨道 : MATLAB Function  TreatAsAtomicUnit=on
  T_gg : Outport
  r_o : Outport  Port=2
  wires:
  [mu] -> Gain/1
  |r_i|/1 -> Pow/1
  Constant/1 -> Pow/2
  卫星对角转动惯量/1 -> Product/1
  地心转轨道/1(r_o) -> r_o/1, Product/2, 叉乘-r_Jr/1
  Product/1 -> 叉乘-r_Jr/2
  Gain/1 -> Divide/2
  Pow/1 -> Divide/1
  Divide/1 -> Product1/2
  叉乘-r_Jr/1 -> Product1/1
  Product1/1 -> T_gg/1
  element/1 -> Bus Selector/1
  Bus Selector/1 -> 地心转轨道/2(i)  "<inc>"
  Bus Selector/4 -> 地心转轨道/5(w)  "<aop>"
  r_i/1 -> 地心转轨道/1(r)
  Bus Selector/2 -> 地心转轨道/3(RA)  "<raan>"
  Bus Selector/3 -> 地心转轨道/4(TA)  "<ta>"

== system satellite3/姿态确定与控制系统/金字塔反作用轮组件 ==
  note: 后续可以调整控制律
  指令力矩 : Inport
  1/eta : Gain  Gain=1/eta
  Abs : Abs  SaturateOnIntegerOverflow=off
  Bus Selector : BusSelector  OutputSignals=wheel1.tau,wheel2.tau,wheel3.tau,wheel4.tau,wheel1.n,wheel2.n,wheel3.n,wheel4.n,wheel1.h,wheel2.h,wheel3.h,wheel4.h
  Gain : Gain  Gain=-1
  Mux : Mux
  Mux1 : Mux
  Mux2 : Mux
  Product : Product
  Scope{,1..3} (4 alike) : Scope
      Scope settings: ActiveDisplayYMinimum=-0.00038870243413452856  ActiveDisplayYMaximum=0.00024212423288498606  DataLoggingVariableName=ScopeData38
      Scope1 settings: ActiveDisplayYMinimum=-0.016121636317304164  ActiveDisplayYMaximum=0.018203231972708345  DataLoggingVariableName=ScopeData39
      Scope2 settings: ActiveDisplayYMinimum=-0.014161413510106281  ActiveDisplayYMaximum=0.061334227613623012  DataLoggingVariableName=ScopeData40
      Scope3 settings: ActiveDisplayYMinimum=-1.9450848600943162E-5  ActiveDisplayYMaximum=1.879321234138711E-5  DataLoggingVariableName=ScopeData28
  Sum of Elements : Sum  Inputs=+
  分配矩阵 : Gain  Gain=K_w  Multiplication=Matrix(K*u)
  反作用轮组件 : Subsystem
  安装 : Gain  Gain=-A_w  Multiplication=Matrix(K*u)
  安装矩阵 : Gain  Gain=A_w  Multiplication=Matrix(K*u)
  简化反作用轮组件 : StateSpace  Commented=on  A=A_mw  B=B_mw  C=C_mw  D=zeros(4,4)  InitialCondition=0
  饱和标志 : Subsystem
  反作用力矩 : Outport
  轮角动量 : Outport  Port=2
  轮功耗 : Outport  Port=3
  wheel : Outport  Port=4
  指令退饱和力矩 : Outport  Port=5
  wires:
  Product/1 -> Abs/1
  安装/1 -> 反作用力矩/1
  分配矩阵/1 -> 简化反作用轮组件/1, Scope3/1, 反作用轮组件/1(指令力矩)
  指令力矩/1 -> Gain/1
  Abs/1 -> Sum of Elements/1
  Sum of Elements/1 -> 1/eta/1
  1/eta/1 -> Scope2/1, 轮功耗/1
  反作用轮组件/1(Wheel) -> wheel/1, Bus Selector/1
  Bus Selector/5 -> Mux1/1  "<n>"
  Bus Selector/6 -> Mux1/2  "<n>"
  Bus Selector/7 -> Mux1/3  "<n>"
  Bus Selector/8 -> Mux1/4  "<n>"
  Mux/1 -> Scope/1, Product/1, 安装/1
  Mux1/1 -> Scope1/1, Product/2
  Bus Selector/1 -> Mux/1  "<tau>"
  Bus Selector/2 -> Mux/2  "<tau>"
  Bus Selector/3 -> Mux/3  "<tau>"
  Bus Selector/4 -> Mux/4  "<tau>"
  Bus Selector/9 -> Mux2/1  "<h>"
  Bus Selector/10 -> Mux2/2  "<h>"
  Bus Selector/11 -> Mux2/3  "<h>"
  Bus Selector/12 -> Mux2/4  "<h>"
  Mux2/1 -> 安装矩阵/1
  安装矩阵/1 -> 饱和标志/1(H), 轮角动量/1
  Gain/1 -> 分配矩阵/1
  饱和标志/1(指令退饱和力矩) -> 指令退饱和力矩/1

== system satellite3/推进子系统/化推 ==
  prop_on : Inport
  thrust_on : Inport  Port=2
  Constant : Constant  Value=D_thr
  Logical Operator : Logic  Inputs=3  AllPortsSameDT=off  OutDataTypeStr=boolean
  PWM : simulink/Discontinuities/PWM  DisableCoverage=on  Period=T_thr  InitialDelay=0  DisallowZeroDutyCycle=off  RunAtFixedTimeIntervals=on  SampleTime=0.1
  Product : Product
  Transfer Fcn1 : TransferFcn  Denominator=[tau_thr 1]
  div_mdot : Product  Inputs=/*
  left_m : Integrator  InitialCondition=m0
  neg_mdot : Gain  Gain=-1
  sat_m : Saturate  UpperLimit=m0  LowerLimit=0
  推力 : Constant  Value=T_nominal
  推力故障 : Subsystem
  比冲*重力加速度 : Constant  Value=Isp*g0
  燃料约束 : RelationalOperator  Operator=>  OutDataTypeStr=boolean  RndMeth=Simplest  InputSameDT=off
  输出推力 : Switch  Criteria=u2 > Threshold  Threshold=0.5  SaturateOnIntegerOverflow=off  InputSameDT=off
  T_act : Outport
  left_fuel : Outport  Port=2
  wires:
  prop_on/1 -> Logical Operator/1  "电"
  thrust_on/1 -> Logical Operator/2  "推"
  neg_mdot/1 -> left_m/1
  比冲*重力加速度/1 -> div_mdot/1
  div_mdot/1 -> neg_mdot/1
  Logical Operator/1 -> 输出推力/2
  输出推力/1 -> Product/1  "T_act"
  [zero] -> 燃料约束/2
  left_m/1 -> sat_m/1
  燃料约束/1 -> Logical Operator/3  "工质"
  [zero] -> 输出推力/3
  sat_m/1 -> left_fuel/1, 燃料约束/1
  推力/1 -> 输出推力/1
  Constant/1 -> PWM/1
  Product/1 -> 推力故障/1(原值)
  推力故障/1(故障值) -> div_mdot/2, T_act/1
  PWM/1 -> Product/2

== system satellite3/推进子系统/向量模长-v ==
  u1 : Inport
  u2 : Inport  Port=2
  u3 : Inport  Port=3
  Add : Sum  Inputs=+++
  Sqrt : Sqrt
  Square : Math  Operator=square
  Square1 : Math  Operator=square
  Square2 : Math  Operator=square
  |u| : Outport
  wires:
  u1/1 -> Square/1
  u2/1 -> Square1/1
  u3/1 -> Square2/1
  Square/1 -> Add/1
  Square1/1 -> Add/2
  Square2/1 -> Add/3
  Add/1 -> Sqrt/1
  Sqrt/1 -> |u|/1

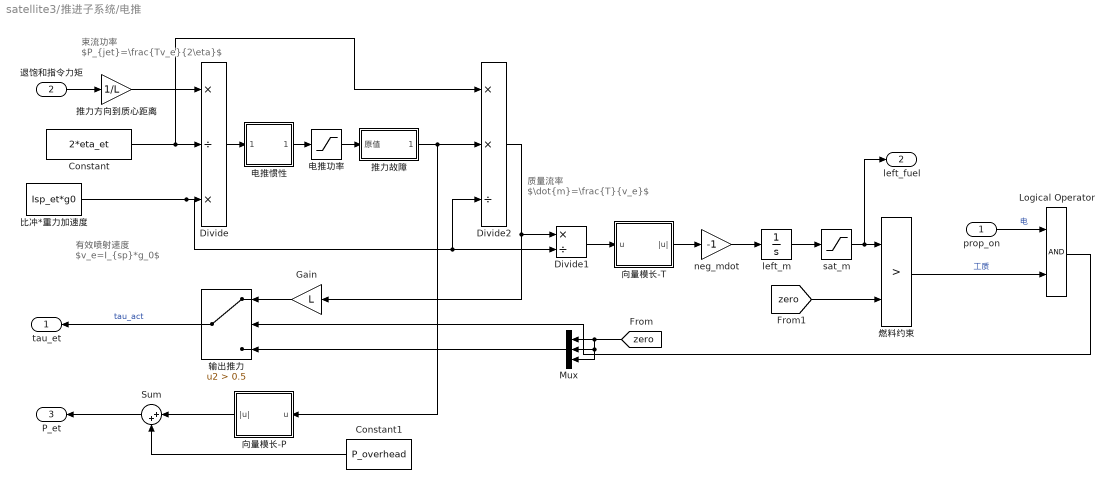
== system satellite3/推进子系统/电推 ==
  note: 质量流率 $\dot{m}=\frac{T}{v_e}$
  note: 束流功率 $P_{jet}=\frac{Tv_e}{2\eta}$
  note: 有效喷射速度 $v_e=I_{sp}*g_0$
  prop_on : Inport
  退饱和指令力矩 : Inport  Port=2
  Constant : Constant  Value=2*eta_et
  Constant1 : Constant  Value=P_overhead
  Divide : Product  Inputs=*/*  OutDataTypeStr=Inherit: Same as first input
  Divide1 : Product  Inputs=*/
  Divide2 : Product  Inputs=**/
  Gain : Gain  Gain=L
  Logical Operator : Logic  AllPortsSameDT=off  OutDataTypeStr=boolean
  Mux : Mux  Inputs=3
  Sum : Sum  Inputs=|++
  left_m : Integrator  InitialCondition=m0_et
  neg_mdot : Gain  Gain=-1
  sat_m : Saturate  UpperLimit=m0_et  LowerLimit=0
  向量模长-P : Subsystem
  向量模长-T : Subsystem
  推力故障 : Subsystem
  推力方向到质心距离 : Gain  Gain=1/L
  比冲*重力加速度 : Constant  Value=Isp_et*g0
  燃料约束 : RelationalOperator  Operator=>  OutDataTypeStr=boolean  RndMeth=Simplest  InputSameDT=off
  电推功率 : Saturate  UpperLimit=P_et_max  LowerLimit=0
  电推惯性 : Subsystem
  输出推力 : Switch  Criteria=u2 > Threshold  Threshold=0.5  SaturateOnIntegerOverflow=off  InputSameDT=off
  tau_et : Outport
  left_fuel : Outport  Port=2
  P_et : Outport  Port=3
  wires:
  燃料约束/1 -> Logical Operator/2  "工质"
  prop_on/1 -> Logical Operator/1  "电"
  比冲*重力加速度/1 -> Divide2/3, Divide1/2, Divide/3
  [zero] -> Mux/3, Mux/2, Mux/1
  输出推力/1 -> tau_et/1  "tau_act"
  Logical Operator/1 -> 输出推力/2
  [zero] -> 燃料约束/2
  left_m/1 -> sat_m/1
  sat_m/1 -> left_fuel/1, 燃料约束/1
  neg_mdot/1 -> left_m/1
  Divide1/1 -> 向量模长-T/1(u)
  退饱和指令力矩/1 -> 推力方向到质心距离/1
  推力方向到质心距离/1 -> Divide/1
  Constant/1 -> Divide2/1, Divide/2
  Divide/1 -> 电推惯性/1(指令)
  电推功率/1 -> 推力故障/1(原值)
  Divide2/1 -> Gain/1, Divide1/1
  Sum/1 -> P_et/1
  Constant1/1 -> Sum/2
  Mux/1 -> 输出推力/3
  Gain/1 -> 输出推力/1
  电推惯性/1(实际) -> 电推功率/1
  向量模长-T/1(|u|) -> neg_mdot/1
  向量模长-P/1(|u|) -> Sum/1
  推力故障/1(故障值) -> 向量模长-P/1(u), Divide2/2

== system satellite3/测控子系统/ECEF2ECI ==
  t : Inport
  Add2 : Sum
  Constant : Constant  Value=earth_theta0
  Constant2 : Constant  Value=sta_vec
  Cos : Trigonometry  Operator=cos
  Gain : Gain  Gain=omegaE
  Gain1 : Gain  Gain=-1
  Mux : Mux  Inputs=3
  Mux1 : Mux  Inputs=3
  Mux2 : Mux  Inputs=3
  Product : Product  Multiplication=Matrix(*)
  Sin : Trigonometry
  Vector Concatenate : Concatenate  NumInputs=3  Mode=Multidimensional array  ConcatenateDimension=2
  eci : Outport
  wires:
  Constant/1 -> Add2/2
  Add2/1 -> Sin/1, Cos/1
  t/1 -> Gain/1
  Cos/1 -> Mux/1, Mux1/2
  Gain/1 -> Add2/1
  Sin/1 -> Mux1/1, Gain1/1
  [zero] -> Mux2/2, Mux2/1, Mux1/3, Mux/3
  [one] -> Mux2/3
  Mux1/1 -> Vector Concatenate/2
  Mux/1 -> Vector Concatenate/1
  Mux2/1 -> Vector Concatenate/3
  Vector Concatenate/1 -> Product/1
  Constant2/1 -> Product/2
  Product/1 -> eci/1
  Gain1/1 -> Mux/2

== system satellite3/测控子系统/ECEF2ENU ==
  ecef : Inport
  Constant : Constant  Value=sta_lat
  Constant1 : Constant  Value=sta_lon
  Cos : Trigonometry  Operator=cos
  Cos1 : Trigonometry  Operator=cos
  Gain : Gain  Gain=-1
  Gain1 : Gain  Gain=-1
  Mux : Mux  Inputs=3
  Mux1 : Mux  Inputs=3
  Mux2 : Mux  Inputs=3
  Product : Product  Multiplication=Matrix(*)
  Product{1..4} (4 alike) : Product
  Sin : Trigonometry
  Sin1 : Trigonometry
  Vector Concatenate : Concatenate  NumInputs=3  Mode=Multidimensional array  ConcatenateDimension=2
  enu : Outport
  wires:
  Constant/1 -> Cos/1, Sin/1
  Vector Concatenate/1 -> Product/1
  ecef/1 -> Product/2
  Product/1 -> enu/1
  Constant1/1 -> Sin1/1, Cos1/1
  Gain/1 -> Mux/1
  Cos1/1 -> Mux/2, Product1/2, Product3/1
  Mux/1 -> Vector Concatenate/1
  Mux1/1 -> Vector Concatenate/2
  Mux2/1 -> Vector Concatenate/3
  [zero] -> Mux/3
  Product1/1 -> Mux1/1
  Sin/1 -> Mux2/3, Gain1/1
  Gain1/1 -> Product2/1, Product1/1
  Product2/1 -> Mux1/2
  Sin1/1 -> Product4/2, Product2/2, Gain/1
  Cos/1 -> Product4/1, Product3/2, Mux1/3
  Product3/1 -> Mux2/1
  Product4/1 -> Mux2/2

== system satellite3/测控子系统/ECI2ECEF ==
  t : Inport
  In1 : Inport  Port=2
  Add2 : Sum
  Constant : Constant  Value=earth_theta0
  Cos : Trigonometry  Operator=cos
  Gain : Gain  Gain=omegaE
  Gain1 : Gain  Gain=-1
  Mux : Mux  Inputs=3
  Mux1 : Mux  Inputs=3
  Mux2 : Mux  Inputs=3
  Product : Product  Multiplication=Matrix(*)
  Sin : Trigonometry
  Vector Concatenate : Concatenate  NumInputs=3  Mode=Multidimensional array  ConcatenateDimension=2
  ecef : Outport
  wires:
  Sin/1 -> Mux/2, Gain1/1
  Product/1 -> ecef/1
  In1/1 -> Product/2
  Vector Concatenate/1 -> Product/1
  Mux2/1 -> Vector Concatenate/3
  Mux/1 -> Vector Concatenate/1
  Mux1/1 -> Vector Concatenate/2
  [one] -> Mux2/3
  [zero] -> Mux/3, Mux1/3, Mux2/1, Mux2/2
  Gain/1 -> Add2/1
  Cos/1 -> Mux1/2, Mux/1
  t/1 -> Gain/1
  Add2/1 -> Cos/1, Sin/1
  Constant/1 -> Add2/2
  Gain1/1 -> Mux1/1

== system satellite3/测控子系统/模长 ==
  u1 : Inport
  u2 : Inport  Port=2
  Add : Sum  Inputs=2
  Sqrt : Sqrt
  Square : Math  Operator=square
  Square1 : Math  Operator=square
  |u| : Outport
  wires:
  Sqrt/1 -> |u|/1
  Add/1 -> Sqrt/1
  Square1/1 -> Add/2
  Square/1 -> Add/1
  u2/1 -> Square1/1
  u1/1 -> Square/1

== system satellite3/测控子系统/测距 ==
  u : Inport
  Add : Sum  Inputs=3
  Demux : Demux  Outputs=3
  Sqrt : Sqrt
  Square : Math  Operator=square
  Square1 : Math  Operator=square
  Square2 : Math  Operator=square
  |u| : Outport
  wires:
  Demux/1 -> Square/1
  Demux/2 -> Square1/1
  Demux/3 -> Square2/1
  Square/1 -> Add/1
  Square1/1 -> Add/2
  Square2/1 -> Add/3
  Add/1 -> Sqrt/1
  Sqrt/1 -> |u|/1
  u/1 -> Demux/1

== system satellite3/测控子系统/视线角标志 ==
  r : Inport
  u : Inport  Port=2
  余弦夹角 : Subsystem
  小于最大视角 : RelationalOperator  OutDataTypeStr=boolean  RndMeth=Simplest  InputSameDT=off
  最大视线角 : Constant  Value=cos_g_max
  Vizlit : Outport
  wires:
  最大视线角/1 -> 小于最大视角/2
  r/1 -> 余弦夹角/1(u1)
  余弦夹角/1(cos(γ)) -> 小于最大视角/1
  u/1 -> 余弦夹角/2(u2)
  小于最大视角/1 -> Vizlit/1

== system satellite3/环境与动力学子系统/J2000模型 ==
  球心距 : Inport
  t : Inport  Port=2
  r_sc : Inport  Port=3
  AND : Logic  AllPortsSameDT=off  OutDataTypeStr=boolean
  Constant : Constant  Value=utc0_jd
  Divide : Product  Inputs=/*
  Dot Product : DotProduct  OutDataTypeStr=Inherit: Inherit via internal rule
  J2000_r_sun : MATLAB Function  TreatAsAtomicUnit=on
  NOT : Logic  Operator=NOT  AllPortsSameDT=off  OutDataTypeStr=boolean
  Relational Operator : RelationalOperator  OutDataTypeStr=boolean  RndMeth=Simplest  InputSameDT=off
  Relational Operator1 : RelationalOperator  Operator=<=  OutDataTypeStr=boolean  RndMeth=Simplest  InputSameDT=off
  Scope{,1..3} (4 alike) : Scope
      Scope settings: ActiveDisplayYMinimum=-1  ActiveDisplayYMaximum=1  DataLoggingVariableName=ScopeData12
      Scope1 settings: DataLoggingVariableName=ScopeData13
      Scope2 settings: ActiveDisplayYMinimum=-1.0981847494910826  ActiveDisplayYMaximum=0.43977554521583484  DataLoggingVariableName=ScopeData15
      Scope3 settings: ActiveDisplayYMinimum=-1  ActiveDisplayYMaximum=1  DataLoggingVariableName=ScopeData16
  Square : Math  Operator=square
  Square1 : Math  Operator=square
  Sum : Sum  Inputs=|-+
  Sum1 : Sum  Inputs=|+-
  rho : Sqrt
  向量模长-r_ss : Subsystem
  地球半径 : Constant  Value=Re
  日照标志 : Outport
  hat_r_ss : Outport  Port=2
  wires:
  t/1 -> J2000_r_sun/1(t)
  Constant/1 -> J2000_r_sun/2(utc0_jd)
  J2000_r_sun/2(s_hat) -> Scope2/1, Dot Product/2
  r_sc/1 -> Sum1/2, Scope3/1, Dot Product/1
  球心距/1 -> Square/1
  Dot Product/1 -> Relational Operator/2, Square1/1
  Square1/1 -> Sum/1
  Square/1 -> Sum/2
  Sum/1 -> rho/1
  rho/1 -> Relational Operator1/1
  [zero] -> Relational Operator/1
  Relational Operator/1 -> Scope/1, AND/1
  地球半径/1 -> Relational Operator1/2
  Relational Operator1/1 -> Scope1/1, AND/2
  AND/1 -> NOT/1
  NOT/1 -> 日照标志/1
  J2000_r_sun/1(r_sun_GCI_km) -> Sum1/1
  Sum1/1 -> Divide/2, 向量模长-r_ss/1(u)
  向量模长-r_ss/1(|u|) -> Divide/1
  Divide/1 -> hat_r_ss/1

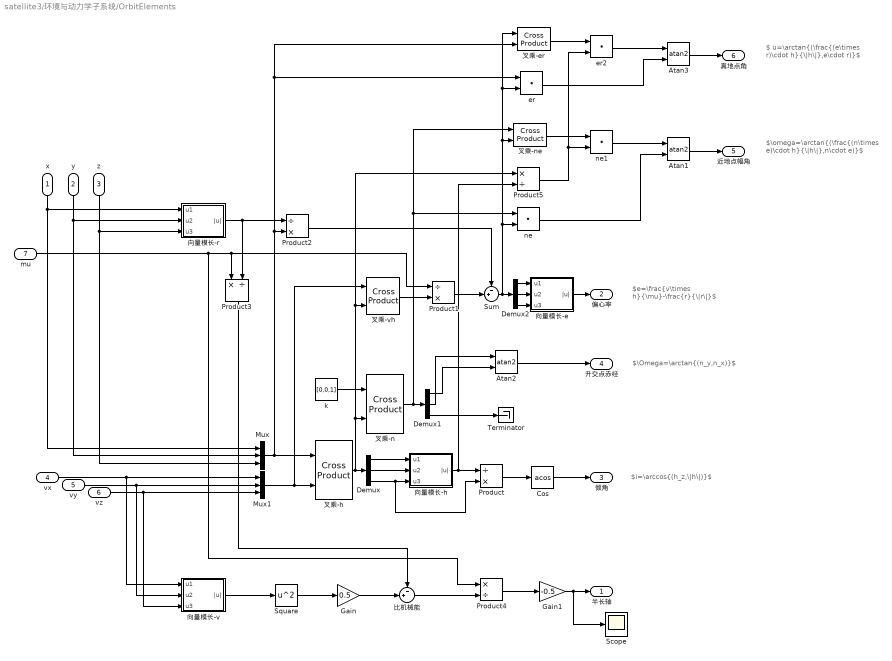
== system satellite3/环境与动力学子系统/OrbitElements ==
  note: $i=\arccos{(h_z,\|h\|)}$
  note: $\Omega=\arctan{(n_y,n_x)}$
  note: $e=\frac{v\times h}{\mu}-\frac{r}{\|r\|}$
  note: $\nu=\arctan{(\frac{(e\times r)\cdot h}{\|h\|},e\cdot r)}$
  note: $\omega=\arctan{(\frac{(n\times e)\cdot h}{\|h\|},n\cdot e)}$
  x : Inport
  y : Inport  Port=2
  z : Inport  Port=3
  vx : Inport  Port=4
  vy : Inport  Port=5
  vz : Inport  Port=6
  mu : Inport  Port=7
  Atan1 : Trigonometry  Operator=atan2
  Atan2 : Trigonometry  Operator=atan2
  Atan3 : Trigonometry  Operator=atan2
  Cos : Trigonometry  Operator=acos
  Demux : Demux  Outputs=3
  Demux1 : Demux  Outputs=3
  Demux2 : Demux  Outputs=3
  Gain : Gain  Gain=0.5
  Gain1 : Gain  Gain=-0.5
  Mux : Mux  Inputs=3
  Mux1 : Mux  Inputs=3
  Product : Product  Inputs=/*
  Product1 : Product  Inputs=/*
  Product2 : Product  Inputs=/*
  Product3 : Product  Inputs=*/
  Product4 : Product  Inputs=*/
  Product5 : Product  Inputs=*/
  Scope : Scope
      settings: ActiveDisplayYMinimum=6.9998946769833127E+6  ActiveDisplayYMaximum=6.9999592468459941E+6  DataLoggingVariableName=ScopeData14
  Square : Math  Operator=square
  Sum : Sum  Inputs=-+|
  Terminator : Terminator
  er : DotProduct  OutDataTypeStr=Inherit: Inherit via internal rule
  er2 : DotProduct  OutDataTypeStr=Inherit: Inherit via internal rule
  k : Constant  Value=[0,0,1]
  ne : DotProduct  OutDataTypeStr=Inherit: Inherit via internal rule
  ne1 : DotProduct  OutDataTypeStr=Inherit: Inherit via internal rule
  叉乘-er : matrix_library/Cross Product
  叉乘-h : matrix_library/Cross Product
  叉乘-n : matrix_library/Cross Product
  叉乘-ne : matrix_library/Cross Product
  叉乘-vh : matrix_library/Cross Product
  向量模长-e : Subsystem
  向量模长-h : Subsystem
  向量模长-r : Subsystem
  向量模长-v : Subsystem
  比机械能 : Sum  Inputs=-+|
  半长轴 : Outport
  偏心率 : Outport  Port=2
  倾角 : Outport  Port=3
  升交点赤经 : Outport  Port=4
  近地点幅角 : Outport  Port=5
  真地点角 : Outport  Port=6
  wires:
  Product/1 -> Cos/1
  向量模长-h/1(|u|) -> Product/1, Product5/2
  Demux/2 -> 向量模长-h/2(u2)
  z/1 -> Mux/3, 向量模长-r/3(u3)
  vx/1 -> Mux1/1, 向量模长-v/1(u1)
  y/1 -> Mux/2, 向量模长-r/2(u2)
  vy/1 -> 向量模长-v/2(u2), Mux1/2
  x/1 -> Mux/1, 向量模长-r/1(u1)
  vz/1 -> Mux1/3, 向量模长-v/3(u3)
  Mux/1 -> er/1, 叉乘-er/2, Product2/2, 叉乘-h/1
  Demux/1 -> 向量模长-h/1(u1)
  Mux1/1 -> 叉乘-h/2, 叉乘-vh/1
  Demux/3 -> Product/2, 向量模长-h/3(u3)
  Cos/1 -> 倾角/1
  叉乘-h/1 -> Product5/1, 叉乘-vh/2, 叉乘-n/2, Demux/1
  叉乘-n/1 -> ne/1, 叉乘-ne/1, Demux1/1
  k/1 -> 叉乘-n/1
  Demux1/1 -> Atan2/2
  Demux1/2 -> Atan2/1
  Demux1/3 -> Terminator/1
  Atan2/1 -> 升交点赤经/1
  叉乘-vh/1 -> Product1/2
  mu/1 -> Product4/1, Product3/1, Product1/1
  向量模长-r/1(|u|) -> Product3/2, Product2/1
  Product1/1 -> Sum/2
  Product2/1 -> Sum/1
  Demux2/1 -> 向量模长-e/1(u1)
  Demux2/2 -> 向量模长-e/2(u2)
  Demux2/3 -> 向量模长-e/3(u3)
  向量模长-e/1(|u|) -> 偏心率/1
  向量模长-v/1(|u|) -> Square/1
  Square/1 -> Gain/1
  Gain/1 -> 比机械能/2
  Product3/1 -> 比机械能/1
  Product4/1 -> Gain1/1
  比机械能/1 -> Product4/2
  Gain1/1 -> Scope/1, 半长轴/1
  叉乘-ne/1 -> ne1/1
  ne1/1 -> Atan1/1
  ne/1 -> Atan1/2
  Atan1/1 -> 近地点幅角/1
  Sum/1 -> ne/2, er/2, 叉乘-er/1, 叉乘-ne/2, Demux2/1
  叉乘-er/1 -> er2/1
  er2/1 -> Atan3/1
  er/1 -> Atan3/2
  Atan3/1 -> 真地点角/1
  Product5/1 -> er2/2, ne1/2
